simulink model "sys_diagram"  (R2022b)
settings: Solver=VariableStepAuto  StartTime=0.0  StopTime=10.0  RelTol=1e-3
undefined symbols (not defined in the file): G, K, W1, W2
settings Model: Creator=scott  LastModifiedBy=scott

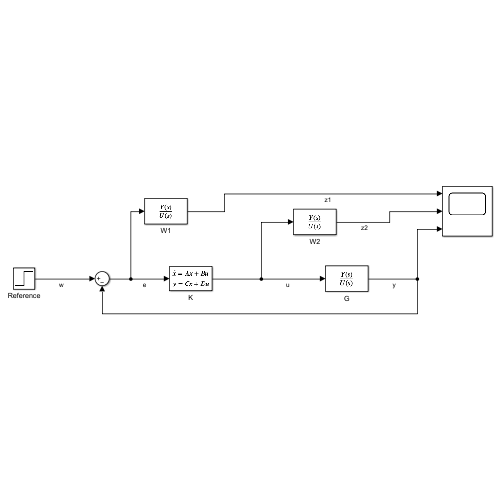
[thumbnail: Simulink's stored preview of the top-level diagram]
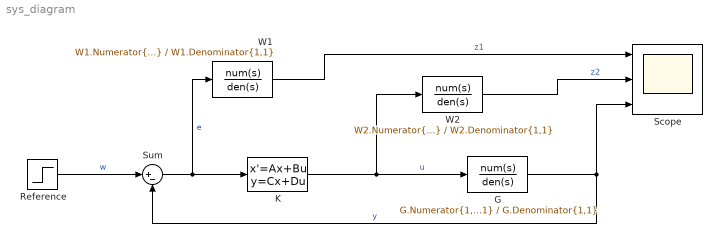
== system sys_diagram ==
  G : TransferFcn  Numerator=G.Numerator{1,1}  Denominator=G.Denominator{1,1}
  K : StateSpace  A=K.A  B=K.B  C=K.C  D=K.D  InitialCondition=0
  Reference : Step  SampleTime=0
  Scope : Scope  NumInputPorts=3
  Sum : Sum  Inputs=|+-
  W1 : TransferFcn  Numerator=W1.Numerator{1,1}  Denominator=W1.Denominator{1,1}  ContinuousStateAttributes='Error weight'
  W2 : TransferFcn  Numerator=W2.Numerator{1,1}  Denominator=W2.Denominator{1,1}  ContinuousStateAttributes='Actuator weight'
  wires:
  K/1 -> G/1, W2/1  "u"
  Sum/1 -> W1/1, K/1  "e"
  Reference/1 -> Sum/1  "w"
  W1/1 -> Scope/1  "z1"
  W2/1 -> Scope/2  "z2"
  G/1 -> Sum/2, Scope/3  "y"
